simulink model "Selector_TestGen13"  (R2017b)
settings: Solver=FixedStepDiscrete  StartTime=0.0  StopTime=10.0  RelTol=1e-3
settings Model: Creator=ktrinh  LastModifiedBy=ktrinh
settings DebuggingCC: ParameterOverflowMsg=none

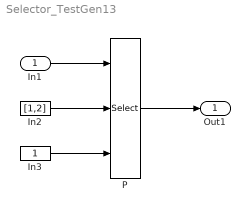
== system Selector_TestGen13 ==
  In1 : Inport  OutDataTypeStr=uint32  PortDimensions=[2 2 2]
  In2 : Constant  Value=[1,2]
  In3 : Constant
  P : Selector  NumberOfDimensions=3  InputPortWidth=3  IndexOptions=Index vector (port),Starting index (dialog),Starting index (port)  Indices=[],1,[]  OutputSizes=,2,2
  Out1 : Outport
  wires:
  In1/1 -> P/1
  In2/1 -> P/2
  In3/1 -> P/3
  P/1 -> Out1/1
